simulink model "autosar_multirunnables_PIL"  (R2018b)
settings: Solver=FixedStepDiscrete  StartTime=0.0  StopTime=200  FixedStep=0.1  MaxStep=.0001  RelTol=1e-3  EnableMultiTasking=on
InitFcn:
  | mbd_s32k_as_consistency_checks(bdroot(gcs));
undefined symbols (not defined in the file): DiscIntNeverNeededParam, LQFP
libraries: mbd_s32k_as_ec_toolbox x1
settings Model: ExtModeAutoUpdateStatusClock=off  Creator=NXP MBDT Team  LastModifiedBy=shivama
settings DataIOCC: ExternalInput=off  InitialState=off  SaveFormat=Array  SaveOutput=off  SignalLogging=off  SaveTime=off
settings OptimizationCC: DefaultParameterBehavior=Inlined  UseDivisionForNetSlopeComputation=on  UseFloatMulNetSlope=on  InlineInvariantSignals=on  EnhancedBackFolding=on  PassReuseOutputArgsAs=Individual arguments  ExpressionDepthLimit=2147483647  ZeroExternalMemoryAtStartup=off  ZeroInternalMemoryAtStartup=off  NoFixptDivByZeroProtection=on  EfficientFloat2IntCast=on  OptimizeBlockOrder=speed  DifferentSizesBufferReuse=on
settings DebuggingCC: SolverPrmCheckMsg=warning  InheritedTsInSrcMsg=none  SingleTaskRateTransMsg=error  SigSpecEnsureSampleTimeMsg=none  ParameterTunabilityLossMsg=error  UnconnectedInputMsg=error  UnconnectedOutputMsg=error  UnconnectedLineMsg=error  BusObjectLabelMismatch=none  UnknownTsInhSupMsg=error  StateNameClashWarn=warning  StrictBusMsg=ErrorOnBusTreatedAsVector  SFUnexpectedBacktrackingDiag=warning  SFNoUnconditionalDefaultTransitionDiag=warning  SFExecutionAtInitializationDiag=none
settings HardwareCC: ProdBitPerPointer=32  ProdBitPerSizeT=32  ProdBitPerPtrDiffT=32  ProdLargestAtomicInteger=Long  ProdLargestAtomicFloat=Double  ProdWordSize=32  ProdHWDeviceType=ARM Compatible->ARM Cortex  TargetIntDivRoundTo=Zero  TargetEndianess=LittleEndian  TargetHWDeviceType=Generic->32-bit Embedded Processor
settings ModelReferenceCC: PropagateSignalLabelsOutOfModel=off
settings SFSimCC: SimUseLocalCustomCode=off  SimParseCustomCode=off  MATLABDynamicMemAlloc=off
settings RTWCC: SystemTargetFile=mbd_s32k_as.tlc  MakeCommand=mbd_s32k_as_make_rtw COPY_MDLREF_INCLUDES=0  TemplateMakefile=mbd_s32k_as.tmf  Description=Model Based Design Autosar Toolbox S32K Code Generation Target  GenerateReport=on  RTWUseLocalCustomCode=off  IncludeHyperlinkInReport=on  LaunchReport=on  CodeExecutionProfiling=on  CodeProfilingSaveOptions=AllData  CodeProfilingInstrumentation=detailed  GenerateTraceInfo=on  GenerateTraceReport=on  GenerateTraceReportSl=on  GenerateTraceReportSf=on  GenerateTraceReportEml=on  GenerateCodeMetricsReport=on
settings CodeAppCC: ForceParamTrailComments=on  IgnoreCustomStorageClasses=off  MaxIdLength=63  OperatorAnnotations=on  SimulinkDataObjDesc=on  SFDataObjDesc=on  CustomSymbolStrGlobalVar=rt$N$M  CustomSymbolStrType=$N$M  CustomSymbolStrFcn=$N$M$F  CustomSymbolStrMacro=$N$M  InsertBlockDesc=on
settings STFCustomTargetCC: MultiwordLength=256  ParMdlRefBuildCompliant=on  CompOptLevelCompliant=on  IncludeMdlTerminateFcn=off  CombineOutputUpdateFcns=on  SuppressErrorStatus=on  ERTCustomFileBanners=on  SupportAbsoluteTime=off  SupportNonFinite=off  SupportComplex=off  SupportContinuousTime=off  SupportNonInlinedSFcns=off  RemoveResetFunc=on  MATLABClassNameForMDSCustomization=Simulink.SoftwareTarget.ERTCustomization  AutosarCompliant=on  LookupTableObjectStructAxisOrder=2,1,3,4,...  LUTObjectStructOrderEvenSpacing=Size,Table,Breakpoints  SystemTargetFile=mbd_s32k_as.tlc
settings ERTTargetCC: ConcurrentExecutionCompliant=off  IncludeMdlTerminateFcn=off  SuppressErrorStatus=on  SupportAbsoluteTime=off  SupportNonFinite=off  SupportComplex=off  ModelStepFunctionPrototypeControlCompliant=off  CPPClassGenCompliant=off  AutosarCompliant=on  UseToolchainInfoCompliant=off  LookupTableObjectStructAxisOrder=2,1,3,4,...  LUTObjectStructOrderEvenSpacing=Size,Table,Breakpoints  InlinedParameterPlacement=NonHierarchical  ERTSrcFileBannerTemplate=mbd_ert_code_template.cgt  ERTHdrFileBannerTemplate=mbd_ert_code_template.cgt  ERTDataSrcFileTemplate=mbd_ert_code_template.cgt  ERTDataHdrFileTemplate=mbd_ert_code_template.cgt  ERTCustomFileTemplate=example_file_process.tlc
settings ConfigComp: CovMetricSettings=dw  CovHtmlReporting=on  CovSaveCumulativeToWorkspaceVar=on  CovSaveSingleToWorkspaceVar=on  CovExternalEMLEnable=off

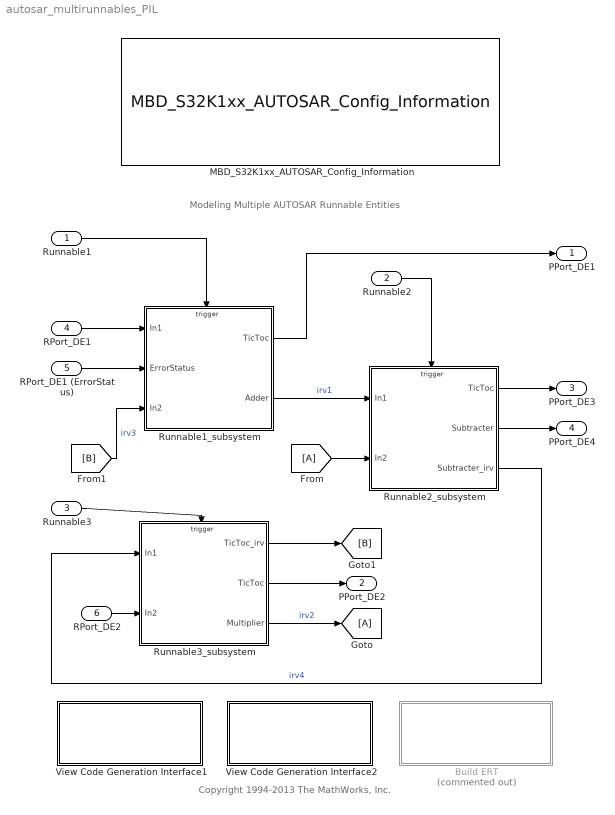
== system autosar_multirunnables_PIL ==
  note: Modeling Multiple AUTOSAR Runnable Entities
  note: Copyright 1994-2013 The MathWorks, Inc.
  Runnable1 : Inport  PortDimensions=1  SampleTime=1  OutputFunctionCall=on
  Runnable2 : Inport  Port=2  PortDimensions=1  SampleTime=1  OutputFunctionCall=on
  Runnable3 : Inport  Port=3  PortDimensions=1  SampleTime=10  OutputFunctionCall=on
  RPort_DE1 : Inport  Port=4  OutDataTypeStr=double  PortDimensions=1
  RPort_DE1 (ErrorStatus) : Inport  Port=5  OutDataTypeStr=uint8  PortDimensions=1
  RPort_DE2 : Inport  Port=6  OutDataTypeStr=double  PortDimensions=2
  Build ERT : Subsystem  Commented=on  mask{attrib_overrides={'RTWCAPIParams','RTWCAPISignals','RTWCAPIStates'}}
      mask prompts: attrib_overrides "List of attributes to preserve (cell of strings):"
      mask help: Enter the attributes of the configuration set that you want preserved. Otherwise, the default configuration script will override your current settings.
      settings: OpenFcn=|
      | try
      |     if ~exist('rtwdemo_ert', 'dir')
      |         disp('Creating working directory rtwdemo_ert')
      |         mkdir('rtwdemo_ert')
      |     end
      |     cd('rtwdemo_ert');
      |     rtwbuilddemomodel('autosar_multirunnables_PIL');
      |     cd('..');
      | catch myException
      |     rethrow(myException);
      | end
      mask Display:
      | disp(['Generate Code Using\n',...
      | 	 'Embedded Coder\n'...
      | 	  '(double-click)'])
  MBD_S32K1xx_AUTOSAR_Config_Information : mbd_s32k_as_ec_toolbox/MBD_S32K1xx_AUTOSAR_Config_Information  mbdt_ver=0  disp_str=|  config_params=[]  mcu_target_name=S32K144  mcu_target_package=48-LQFP  mcu_target_sram_size=64KB  mcu_system_clock_freq=80  mcu_xtal_freq=External 8  mcu_steptick_timer=LPIT Channel 0  mcu_steptick_prio=15  ds_import_enable=on  target_compiler=GCC  target_memory=FLASH  gcc_target_compile_opts=-mcpu=cortex-m4 -mthumb -mfloat-abi=hard -mfpu=fpv4-sp-d16 -O1 -g -gstrict-dwarf  gcc_target_assemble_opts=-mcpu=cortex-m4 -mthumb -mfloat-abi=hard -mfpu=fpv4-sp-d16 -g  gcc_target_link_opts=-mcpu=cortex-m4 -mthumb -mfloat-abi=hard -mfpu=fpv4-sp-d16  gcc_target_default_lcf=on  gcc_target_user_lcf=S32K144_64_flash.ld  ghs_target_compile_opts=-cpu=cortexm4f -thumb -fpu=vfpv4_d16 -fsingle -Ogeneral -Wundef -Wimplicit-int -Wshadow -Wtrigraphs --no_commons --gnu_asm -gnu99 -gdwarf-2 -G  ghs_target_assemble_opts=-cpu=cortexm4f -fpu=vfpv4_d16  ghs_target_link_opts=-cpu=cortexm4f -thumb -fpu=vfpv4_d16  ghs_target_default_lcf=on  ghs_target_user_lcf=S32K144_64_flash.ld  iar_target_compile_opts=--cpu=Cortex-M4F --thumb --fpu=VFPv4_sp -Ol -e --debug --dlib_config normal  iar_target_assemble_opts=--cpu Cortex-M4F --thumb --fpu VFPv4_sp  iar_target_link_opts=--no_exceptions --vfe --inline  iar_target_default_lcf=on  iar_target_user_lcf=S32K144_64_flash.icf  pil_download_enable=on  rbl_download_enable=off  rbl_start_delay=5000  rbl_download_interface=OpenSDA  rbl_restart_request=off  rbl_com_port=Custom  rbl_com_port_custom=COM1  pil_download_rate=38400  pil_opensda_drive=Custom  pil_opensda_drive_custom=D  pil_uart_instance=1  pil_uart_rx=PTC6: [LPUART1_RX | Receive]  pil_uart_tx=PTC7: [LPUART1_TX | Transmit]  Profile_PcrCheckEnDis=on  ConfigParams_PcrCheckEnDis=off  ModelRef_PcrCheckEnDis=on
      | Target : S32K144-64KB_SRAM
      | Package : 100-pin
      | System clock : 80 MHz
      | XTAL clock : External 8 MHz
      | Compiler : IAR
      | Target Type : FLASH
      | Download Code after build : off
      | Step Tick Interrupt Priority : 15
  Runnable1_subsystem : Subsystem  Tag=DoNotProfile  TreatAsAtomicUnit=on  RTWFcnName=foo
  Runnable2_subsystem : Subsystem  Tag=DoNotProfile  TreatAsAtomicUnit=on  RTWFcnName=foo
  Runnable3_subsystem : Subsystem  Tag=DoNotProfile  TreatAsAtomicUnit=on  RTWFcnName=foo
  View Code Generation Interface1 : Subsystem
      settings: OpenFcn=autosar_ui_launch('autosar_multirunnables_PIL')
      mask Display: disp('Configure Model\nAs AUTOSAR\nSoftware Component\n(double-click)')
  View Code Generation Interface2 : Subsystem
      settings: OpenFcn=|
      | dlg = slCfgPrmDlg(bdroot,'Open');
      | dlg = slCfgPrmDlg(bdroot,'TurnToPage','Code Generation/AUTOSAR Code Generation Options'); clear dlg;
      mask Display: disp('View AUTOSAR\nCode Generation\nOptions\n(double-click)')
  PPort_DE1 : Outport  OutDataTypeStr=int8  PortDimensions=1
  PPort_DE2 : Outport  Port=2  OutDataTypeStr=int8  PortDimensions=1
  PPort_DE3 : Outport  Port=3  OutDataTypeStr=int8  PortDimensions=2
  PPort_DE4 : Outport  Port=4  OutDataTypeStr=double  PortDimensions=1
  wires:
  [B] -> Runnable1_subsystem/3(In2)  "irv3"
  Runnable3_subsystem/1(TicToc_irv) -> [B]
  [A] -> Runnable2_subsystem/2(In2)
  Runnable3_subsystem/3(Multiplier) -> [A]  "irv2"
  RPort_DE1 (ErrorStatus)/1 -> Runnable1_subsystem/2(ErrorStatus)
  Runnable2_subsystem/2(Subtracter) -> PPort_DE4/1
  RPort_DE1/1 -> Runnable1_subsystem/1(In1)
  Runnable2/1 -> Runnable2_subsystem/Trigger
  Runnable1_subsystem/1(TicToc) -> PPort_DE1/1
  Runnable2_subsystem/1(TicToc) -> PPort_DE3/1
  Runnable3_subsystem/2(TicToc) -> PPort_DE2/1
  Runnable1/1 -> Runnable1_subsystem/Trigger
  Runnable1_subsystem/2(Adder) -> Runnable2_subsystem/1(In1)  "irv1"
  Runnable2_subsystem/3(Subtracter_irv) -> Runnable3_subsystem/1(In1)  "irv4"
  RPort_DE2/1 -> Runnable3_subsystem/2(In2)
  Runnable3/1 -> Runnable3_subsystem/Trigger

== system autosar_multirunnables_PIL/Build ERT ==

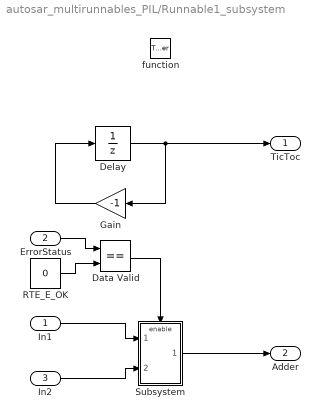
== system autosar_multirunnables_PIL/Runnable1_subsystem ==
  In1 : Inport
  ErrorStatus : Inport  Port=2
  In2 : Inport  Port=3
  function : TriggerPort  TriggerType=function-call  VariantControl=(inherit)  SampleTimeType=periodic  SampleTime=-1
  Data Valid : RelationalOperator  Operator===  OutDataTypeStr=boolean  RndMeth=Nearest
  Delay : UnitDelay  InitialCondition=1  SampleTime=-1
  Gain : Gain  Gain=-1  OutDataTypeStr=fixdt(1,8,0)
  RTE_E_OK : Constant  Value=0
  Subsystem : Subsystem
  TicToc : Outport  InitialOutput=0
  Adder : Outport  Port=2  InitialOutput=0
  wires:
  RTE_E_OK/1 -> Data Valid/2
  ErrorStatus/1 -> Data Valid/1
  Data Valid/1 -> Subsystem/Enable
  In2/1 -> Subsystem/2(In2)
  In1/1 -> Subsystem/1(In1)
  Delay/1 -> Gain/1, TicToc/1
  Gain/1 -> Delay/1
  Subsystem/1(Out1) -> Adder/1

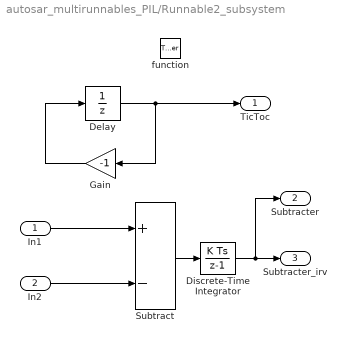
== system autosar_multirunnables_PIL/Runnable2_subsystem ==
  In1 : Inport
  In2 : Inport  Port=2
  function : TriggerPort  TriggerType=function-call  VariantControl=(inherit)  SampleTimeType=periodic  SampleTime=-1
  Delay : UnitDelay  InitialCondition=1  SampleTime=-1
  Discrete-Time Integrator : DiscreteIntegrator  SampleTime=-1  ICPrevOutput=DiscIntNeverNeededParam  ICPrevScaledInput=DiscIntNeverNeededParam
  Gain : Gain  Gain=-1  OutDataTypeStr=fixdt(1,8,0)
  Subtract : Sum  Inputs=+-
  TicToc : Outport  InitialOutput=0
  Subtracter : Outport  Port=2  InitialOutput=0
  Subtracter_irv : Outport  Port=3
  wires:
  Discrete-Time Integrator/1 -> Subtracter/1, Subtracter_irv/1
  Subtract/1 -> Discrete-Time Integrator/1
  Gain/1 -> Delay/1
  Delay/1 -> TicToc/1, Gain/1
  In1/1 -> Subtract/1
  In2/1 -> Subtract/2

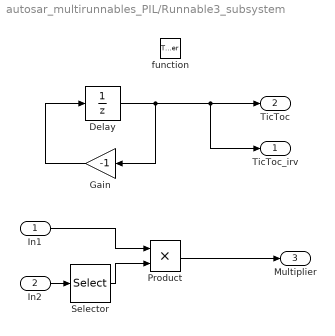
== system autosar_multirunnables_PIL/Runnable3_subsystem ==
  In1 : Inport  OutDataTypeStr=double
  In2 : Inport  Port=2
  function : TriggerPort  TriggerType=function-call  VariantControl=(inherit)  SampleTimeType=periodic  SampleTime=-1
  Delay : UnitDelay  InitialCondition=1  SampleTime=-1
  Gain : Gain  Gain=-1  OutDataTypeStr=fixdt(1,8,0)
  Product : Product  Inputs=**  OutDataTypeStr=Inherit: Same as first input
  Selector : Selector  InputPortWidth=2  IndexOptions=Index vector (dialog)  Indices=1  OutputSizes=1
  TicToc_irv : Outport
  TicToc : Outport  Port=2  InitialOutput=0
  Multiplier : Outport  Port=3  InitialOutput=0
  wires:
  Selector/1 -> Product/2
  Product/1 -> Multiplier/1
  Gain/1 -> Delay/1
  Delay/1 -> TicToc_irv/1, TicToc/1, Gain/1
  In1/1 -> Product/1
  In2/1 -> Selector/1

== system autosar_multirunnables_PIL/View Code Generation Interface1 ==

== system autosar_multirunnables_PIL/View Code Generation Interface2 ==

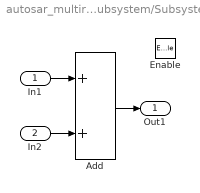
== system autosar_multirunnables_PIL/Runnable1_subsystem/Subsystem ==
  In1 : Inport
  In2 : Inport  Port=2
  Enable : EnablePort
  Add : Sum
  Out1 : Outport
  wires:
  In2/1 -> Add/2
  Add/1 -> Out1/1
  In1/1 -> Add/1
